simulink model "single_particle_model"  (R2024a)
settings: Solver=FixedStepAuto  StartTime=0.0  StopTime=1  FixedStep=0.5  RelTol=1e-3
settings Model: Creator=jagmohan  LastModifiedBy=jagmohan

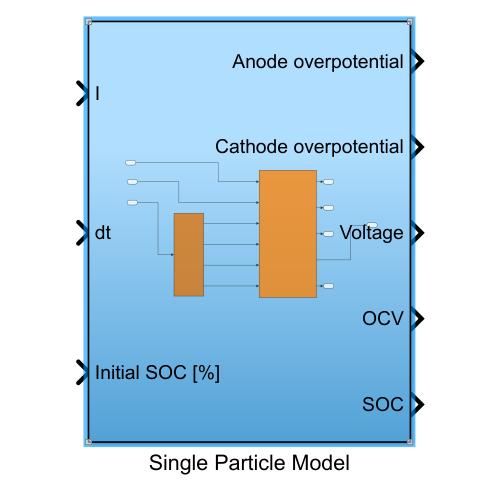
[thumbnail: Simulink's stored preview of the top-level diagram]
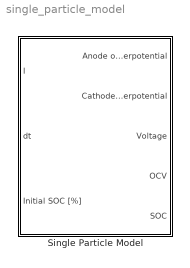
== system single_particle_model ==
  Single Particle Model : Subsystem

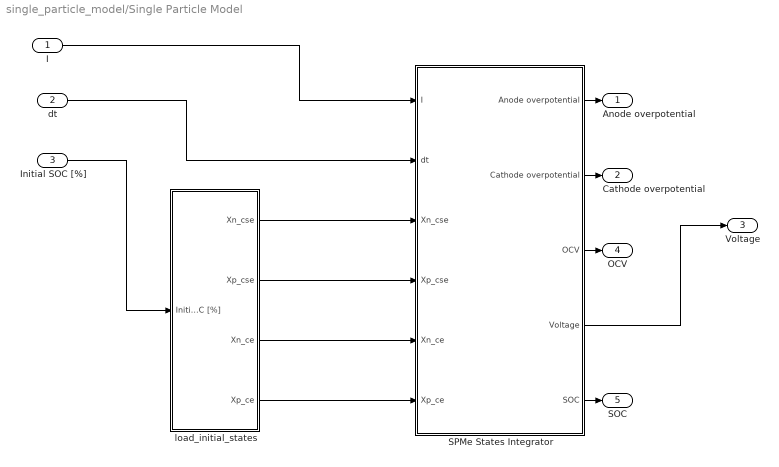
== system single_particle_model/Single Particle Model ==
  I : Inport
  dt : Inport  Port=2
  Initial SOC [%] : Inport  Port=3
  SPMe States Integrator : Subsystem
  load_initial_states : Subsystem
  Anode overpotential : Outport
  Cathode overpotential : Outport  Port=2
  Voltage : Outport  Port=3
  OCV : Outport  Port=4
  SOC : Outport  Port=5
  wires:
  I/1 -> SPMe States Integrator/1(I)
  load_initial_states/1(Xn_cse) -> SPMe States Integrator/3(Xn_cse)
  SPMe States Integrator/3(OCV) -> OCV/1
  SPMe States Integrator/1(Anode overpotential) -> Anode overpotential/1
  load_initial_states/3(Xn_ce) -> SPMe States Integrator/5(Xn_ce)
  load_initial_states/2(Xp_cse) -> SPMe States Integrator/4(Xp_cse)
  SPMe States Integrator/4(Voltage) -> Voltage/1
  load_initial_states/4(Xp_ce) -> SPMe States Integrator/6(Xp_ce)
  SPMe States Integrator/2(Cathode overpotential) -> Cathode overpotential/1
  SPMe States Integrator/5(SOC) -> SOC/1
  Initial SOC [%]/1 -> load_initial_states/1(Initial SOC [%])
  dt/1 -> SPMe States Integrator/2(dt)

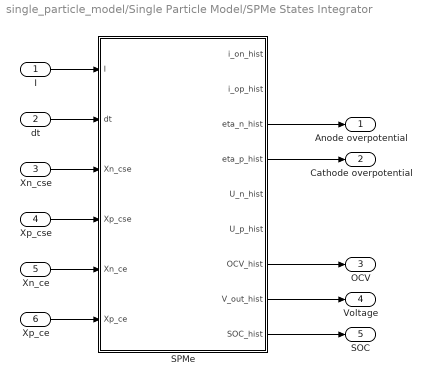
== system single_particle_model/Single Particle Model/SPMe States Integrator ==
  I : Inport
  dt : Inport  Port=2
  Xn_cse : Inport  Port=3
  Xp_cse : Inport  Port=4
  Xn_ce : Inport  Port=5
  Xp_ce : Inport  Port=6
  SPMe : MATLAB Function  TreatAsAtomicUnit=on  mask{num_time_steps=100}
      mask prompts: num_time_steps "Number of time steps"
  Anode overpotential : Outport
  Cathode overpotential : Outport  Port=2
  OCV : Outport  Port=3
  Voltage : Outport  Port=4
  SOC : Outport  Port=5
  wires:
  Xp_ce/1 -> SPMe/6(Xp_ce)
  SPMe/8(V_out_hist) -> Voltage/1
  SPMe/9(SOC_hist) -> SOC/1
  dt/1 -> SPMe/2(dt)
  SPMe/3(eta_n_hist) -> Anode overpotential/1
  SPMe/4(eta_p_hist) -> Cathode overpotential/1
  Xp_cse/1 -> SPMe/4(Xp_cse)
  I/1 -> SPMe/1(I)
  Xn_cse/1 -> SPMe/3(Xn_cse)
  Xn_ce/1 -> SPMe/5(Xn_ce)
  SPMe/7(OCV_hist) -> OCV/1

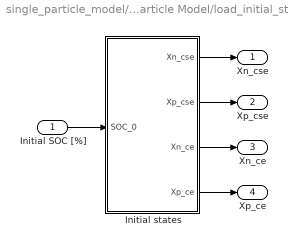
== system single_particle_model/Single Particle Model/load_initial_states ==
  Initial SOC [%] : Inport
  Initial states : MATLAB Function  TreatAsAtomicUnit=on
  Xn_cse : Outport
  Xp_cse : Outport  Port=2
  Xn_ce : Outport  Port=3
  Xp_ce : Outport  Port=4
  wires:
  Initial states/4(Xp_ce) -> Xp_ce/1
  Initial states/3(Xn_ce) -> Xn_ce/1
  Initial states/2(Xp_cse) -> Xp_cse/1
  Initial states/1(Xn_cse) -> Xn_cse/1
  Initial SOC [%]/1 -> Initial states/1(SOC_0)

== matlab function single_particle_model/Single Particle Model/SPMe States Integrator/SPMe ==
  data: i_on_hist output; i_op_hist output; eta_n_hist output; eta_p_hist output; U_n_hist output; U_p_hist output; OCV_hist output; V_out_hist output; SOC_hist output; I input size=1; dt input size=1; Xn_cse input size=3; Xp_cse input size=3; Xn_ce input size=1; Xp_ce input size=1; num_time_steps parameter size=1
function [i_on_hist, i_op_hist, eta_n_hist, eta_p_hist, U_n_hist, U_p_hist, OCV_hist, V_out_hist, SOC_hist] = fcn(I, dt, Xn_cse, Xp_cse, Xn_ce, Xp_ce, num_time_steps)


    %% Define states of the system (persistent variable used since we need to store the previous states)
    
    % persistent Xn_cse Xp_cse Xn_ce Xp_ce
    
    C_bat = 5.032; % [Ah] nominal battery capacity (note: my LGM50T cell in the lab has a capacity of 5.0032 Ah)
    L_n = 85.2e-6; % [m] thickness of negative electrode
    L_sep = 12e-6; % [m] thickness of separator
    L_p = 75.6e-6; % [m] thickness of positive electrode
    R_s_n = 5.86e-6; % [m] radius of solid negative electrode particle
    R_s_p = 5.22e-6; % [m] radius of solid positive electrode particle
    Area_n = 0.1027; % [m^2] negative electrode current collector area
    Area_p = 0.1027; % [m^2] positive electrode current collector area

    % Note: Need to update all epsilon parameters based on the cell
    epsilon_e_n = (0.335+0.25)/2; % [-] active material volume fraction (porosity) of electrolyte in negative electrode
    epsilon_e_sep = 0.47; % [-] active material volume fraction (porosity) of electrolyte in separator
    epsilon_e_p = (0.335+0.25)/2; % [-] active material volume fraction (porosity) of electrolyte in positive electrode

    epsilon_s_n = 0.7374; % [-] active material volume fraction of solid negative electrode
    epsilon_s_p = 0.5758; % [-] active material volume fraction of solid positive electrode    
    t_plus = 0.2594; % [-] transference number

    gamma = 0; % [-] activity coefficient
    k_n = 6.7160e-12; % [(mol/(s*m^2))*(mol/m^3)^(-3*alpha)] reaction rate in negative electrode
    k_p = 3.5446e-11; % [(mol/(s*m^2))*(mol/m^3)^(-3*alpha)] reaction rate in positive electrode
    alpha = 0.5; % [-] charge transfer coefficient (for positive and negative electrodes)
    R_f_n = 0; % [Ohms*m^2] resistivity of SEI layer for negative electrode
    R_f_p = 0; % [Ohms*m^2] resistivity of SEI layer for positive electrode
    R_c = 0; %  [Ohms*m^2] contact resistance (resistance of current collectors and wiring)
    kappa = 0.9487; % [1/Ohms-m] electrolyte conductivity

    % Computed Parameters
    a_s_n = 3*epsilon_s_n/R_s_n; % [1/m] negative electrode specific interfacial surface area
    a_s_p = 3*epsilon_s_p/R_s_p; % [1/m] positive electrode specific interfacial surface area
    epsilon_e = mean([epsilon_e_n,epsilon_e_p]); % [-] uniform active material volume fraction of electrolyte in electrodes (for Pade approximation)
    % Limits
    V_out_max = 4.5; % [V] terminal voltage upper limit
    V_out_min = 2.5; % [V] terminal voltage lower limit
    SOC_max = 1; % [-] SOC upper limit
    SOC_min = 0; % [-] SOC lower limit
    cse_n_max = 33133; % [mol/m^3] max concentration in negative electrode
    cse_p_max = 63104; % [mol/m^3] max concentration in positive electrode
    ce_0 = 1000; % [mol/m^3] Initial concentration of Li in electrolyte
    %Note: Need to update all theta parameters based on the cell
    theta_n_0 = 0.0282; % [-] negative electrode surface stoichiometry when SOC = 0
    theta_n_1 = 0.9014; % [-] negative electrode surface stoichiometry when SOC = 1
    theta_p_0 = 0.9369; % [-] positive electrode surface stoichiometry when SOC = 0
    theta_p_1 = 0.2752; % [-] positive electrode surface stoichiometry when SOC = 1

    R = 8.314472; % [J/mol-K] universal gas constant
    T = 298.15; % [K] cell temperature
    F = 96485.33289; % [C/mol] Faraday constant


    %%% Solid n-electrode
    % Solid n-electrode: Continuous state-space
    A1 = [0 1 0; 0 0 1; 0 -0.00319993130126051 -0.181627042831017];
    B1 = [0; 0; 1];
    C1 = [-1638.19008596954, -206629.172731533, -3583617.74744027];
    D1 = 0;
    % Solid n-electrode: Discrete state-space
    Ad_cse_n = A1*dt + eye(size(A1));
    Bd_cse_n = B1*dt;
    Cd_cse_n = C1;
    Dd_cse_n = D1;

    %%% Solid p-electrode
    % Solid p-electrode: Continuous state-space
    A2 = [0 1 0; 0 0 1; 0 -7.46691503526743e-05 -0.02774474831549747];
    B2 = [0; 0; 1];
    C2 = [-42.9133048003876, -35433.9058946327, -4022988.50574713];
    D2 = 0;
    % Solid p-electrode: Discrete state-space
    Ad_cse_p = A2*dt + eye(size(A2));
    Bd_cse_p = B2*dt;
    Cd_cse_p = C2;
    Dd_cse_p = D2;

    %%% Electrolyte dynamics: n-electrode
    A3 = -0.032484;
    B3 = 1;
    C3 = 3.6891;
    D3 = 0;
    Ad_ce_n = A3*dt + eye(size(A3));
    Bd_ce_n = B3*dt;
    Cd_ce_n = C3;
    Dd_ce_n = D3;

    %%% Electrolyte dynamics: p-electrode
    A4 = -0.033647;
    B4 = 1;
    C4 = 3.9316;
    D4 = 0;
    Ad_ce_p = A4*dt + eye(size(A4));
    Bd_ce_p = B4*dt;
    Cd_ce_p = C4;
    Dd_ce_p = D4;

    % Time array length
    % steps = num_time_steps; % TODO: change it for input current profiles

    %% Preallocate Arrays for Time History
    % num_time_steps = 100;
    i_on_hist = zeros(num_time_steps, 1);
    i_on_hist = zeros(num_time_steps, 1);
    i_op_hist = zeros(num_time_steps, 1);
    eta_n_hist = zeros(num_time_steps, 1);
    eta_p_hist = zeros(num_time_steps, 1);
    U_n_hist = zeros(num_time_steps, 1);
    U_p_hist = zeros(num_time_steps, 1);
    V_out_hist = zeros(num_time_steps, 1);
    SOC_hist = zeros(num_time_steps, 1);
    OCV_hist = zeros(num_time_steps, 1);

    %% Run state space model to get the next states
    
    for t = 1:num_time_steps

        %% Define Inputs to state-space models
        j_n = +I./(Area_n*L_n);   % curren flux at n-electrode: j_n(Li) = I/A*thickness 
        j_p = -I./(Area_p*L_p);   % curren flux at p-electrode: j_p(Li) = -I/A*thickness 
        inp_cse_n = j_n./(F*a_s_n);    % Input for negative electrode
        inp_cse_p = j_p./(F*a_s_p);    % Input for positive electrode
        inp_ce_n = I;  % Input for electrolyte at n-electrode
        inp_ce_p = I;  % Input for electrolyte at p-electrode

        % solid n-electrode
        Xn_cse = Ad_cse_n*(Xn_cse) + Bd_cse_n*inp_cse_n;
        cse_n = Cd_cse_n*(Xn_cse) + Dd_cse_n*inp_cse_n;

        % solid p-electrode
        Xp_cse = Ad_cse_p*Xp_cse + Bd_cse_p*inp_cse_p;
        cse_p = Cd_cse_p*Xp_cse + Dd_cse_p*inp_cse_p;

        % n-electrolyte
        Xn_ce = Ad_ce_n*Xn_ce + Bd_ce_n*inp_ce_n;
        ce_n = Cd_ce_n*Xn_ce + Dd_ce_n*inp_ce_n + ce_0; % ce_0 added to compansate for zero IC

        % p-electrolyte
        Xp_ce = Ad_ce_p*Xp_ce + Bd_ce_p*inp_ce_p;
        ce_p = Cd_ce_p*Xp_ce + Dd_ce_p*inp_ce_p + ce_0;  % ce_0 added to compansate for zero IC 

        % Li intercalation/deintercalation  
        i_on = F*k_n*(ce_0^alpha)*((cse_n_max - cse_n)^alpha)*(cse_n^alpha); % corrected with ce_0
        i_op = F*k_p*(ce_0^alpha)*((cse_p_max - cse_p)^alpha)*(cse_p^alpha); % corrected with ce_0
        zeta_n = j_n/(2*a_s_n*i_on);
        zeta_p = j_p/(2*a_s_p*i_op);
        del_phi_e_con = (2*R*T*(1-t_plus)/F)*(1+gamma)*log(ce_p/ce_n);   

        % Battery terminal voltage and overpotential
        eta_n = (R*T/(alpha*F))*log(zeta_n + sqrt(zeta_n^2 + 1));
        eta_p = (R*T/(alpha*F))*log(zeta_p + sqrt(zeta_p^2 + 1));

        % Open Circuit Potential
        theta_n = cse_n/cse_n_max; % [-] negative electrode surface stoichiometry
        U_n = 1.9793*exp(-39.3631*theta_n)+0.2482...
                -0.0909*tanh(29.8538*(theta_n-0.1234))...
                -0.04478*tanh(14.9159*(theta_n-0.2769))...
                -0.0205*tanh(30.4444*(theta_n-0.6103)); % [V] open circuit potential for negative electrode

        theta_p = cse_p / cse_p_max; % [-] positive electrode surface stoichiometry
        U_p = -0.809*theta_p+4.4875-0.0428*tanh(18.5138*(theta_p-0.5542))-...
                17.7326*tanh(15.789*(theta_p-0.3117))+...
                17.5842*tanh(15.9308*(theta_p-0.312)); % [V] open circuit potential for positive electrode

        % effective resistance
        d_n = L_n; % [m] n-electrode thickness
        d_p = L_p; % [m] p-electrode thickness
        d_sep = L_sep; % [m] separator thickness
        R_omega = R_c/Area_n + R_f_n/(Area_n*d_n*a_s_n) + R_f_p/(Area_p*d_p*a_s_p) + ...
        (d_n + d_p)/(2*Area_n*kappa*epsilon_e^1.5) + (d_sep)/(Area_n*kappa*epsilon_e_sep^1.5);
        
        % Open circuit voltage (OCV)
        OCV = U_p - U_n;

        % Voltage output
        V_out = OCV + del_phi_e_con + eta_p - eta_n - I*R_omega;  

        % SOC
        SOC_n = (theta_n - theta_n_0)/(theta_n_1 - theta_n_0); % [-] SOC from negative electrode surface stoichiometry
        SOC_p = (theta_p - theta_p_0)/(theta_p_1 - theta_p_0); % [-] SOC from positive electrode surface stoichiometry
        SOC = (SOC_n + SOC_p)/2; % [-] mean SOC

        % Store the time history
        i_on_hist(t) = i_on;
        i_op_hist(t) = i_op;
        eta_n_hist(t) = eta_n;
        eta_p_hist(t) = eta_p;
        U_n_hist(t) = U_n;
        U_p_hist(t) = U_p;
        V_out_hist(t) = V_out;
        SOC_hist(t) = SOC;
        OCV_hist(t) = OCV; 

    end

    end

== matlab function single_particle_model/Single Particle Model/load_initial_states/Initial states ==
  data: SOC_0 input size=1; Xn_cse output size=3; Xp_cse output size=3; Xn_ce output size=1; Xp_ce output size=1
function [Xn_cse, Xp_cse, Xn_ce, Xp_ce] = fcn(SOC_0)

    
    % Convert SOC from percentage to fraction
    SOC_0 = SOC_0/100;

    %% Fixed parameters
    
    % Limits
    cse_n_max = 33133; % [mol/m^3] max concentration in negative electrode
    cse_p_max = 63104; % [mol/m^3] max concentration in positive electrode
    %Note: Need to update all theta parameters based on the cell
    theta_n_0 = 0.0282; % [-] negative electrode surface stoichiometry when SOC = 0
    theta_n_1 = 0.9014; % [-] negative electrode surface stoichiometry when SOC = 1
    theta_p_0 = 0.9369; % [-] positive electrode surface stoichiometry when SOC = 0
    theta_p_1 = 0.2752; % [-] positive electrode surface stoichiometry when SOC = 1
    
    %% Initialize state-space model
    
    theta_n = (theta_n_1-theta_n_0)*SOC_0+theta_n_0; % [-] initial negative electrode surface stoichiometry
    theta_p = theta_p_0-(theta_p_0-theta_p_1)*SOC_0; % [-] initial positive electrode surface stoichiometry
    cse_0_n = theta_n*cse_n_max; % [mol/m^3] initial concentration of ions in negative solid electrode
    cse_0_p = theta_p*cse_p_max; % [mol/m^3] initial concentration of ions in positive solid electrode

    cse_n_init = zeros(3,1); 
    cse_n_init(1) = cse_0_n/(-1638.19008596954);
    cse_p_init = zeros(3,1); 
    cse_p_init(1) = cse_0_p/(-42.9133048003876);
    ce_n_init = 0;   % IC for electrolyte at n-electrode
    ce_p_init = 0;   % IC for electrolyte at p-electrode

    %%% Initial conditions
    % n-electrode
    Xn_cse = cse_n_init;      
    % p-electrode 
    Xp_cse = cse_p_init;
    % n-lectrolyte
    Xn_ce = ce_n_init;
    % p-electrolyte
    Xp_ce = ce_p_init;

end
